simulink model "SLAMtester1"  (R2014a)
settings: Solver=FixedStepDiscrete  StartTime=0.0  StopTime=inf  FixedStep=.1  RelTol=1e-3
undefined symbols (not defined in the file): Com1, Com2, Com3, Com4, RGB24, standard
libraries: xpcseriallib x10, speedgoatlib_IO102 x6, slrtlib x4, xpcvideousblib x2, xpcvideoutillib x2, speedgoatlib x1
(part 1 of 2)
settings Model: BufferReuse=off  Creator=wildcat  LastModifiedBy=Villanova ASV
settings SolverCC: EnableConcurrentExecution=on
settings DataIOCC: SignalLoggingSaveFormat=ModelDataLogs
settings OptimizationCC: BlockReduction=off  OptimizeBlockIOStorage=off  BufferReuse=off  GlobalBufferReuse=off  ExpressionFolding=off  LocalBlockOutputs=off
settings DebuggingCC: UnderspecifiedInitializationDetection=Classic  StateNameClashWarn=warning
settings HardwareCC: ProdIntDivRoundTo=Zero  ProdEndianess=LittleEndian  ProdHWDeviceType=Generic->32-bit x86 compatible
settings RTWCC: SystemTargetFile=slrt.tlc  TemplateMakefile=slrt_default_tmf  Description=Simulink Real-Time  ProcessScript=slrt_make_rtw_hook  RTWCompilerOptimization=On
settings SimulinkRealTimeCC: GeneratePreprocessorConditionals=Disable all  EnableShiftOperators=on

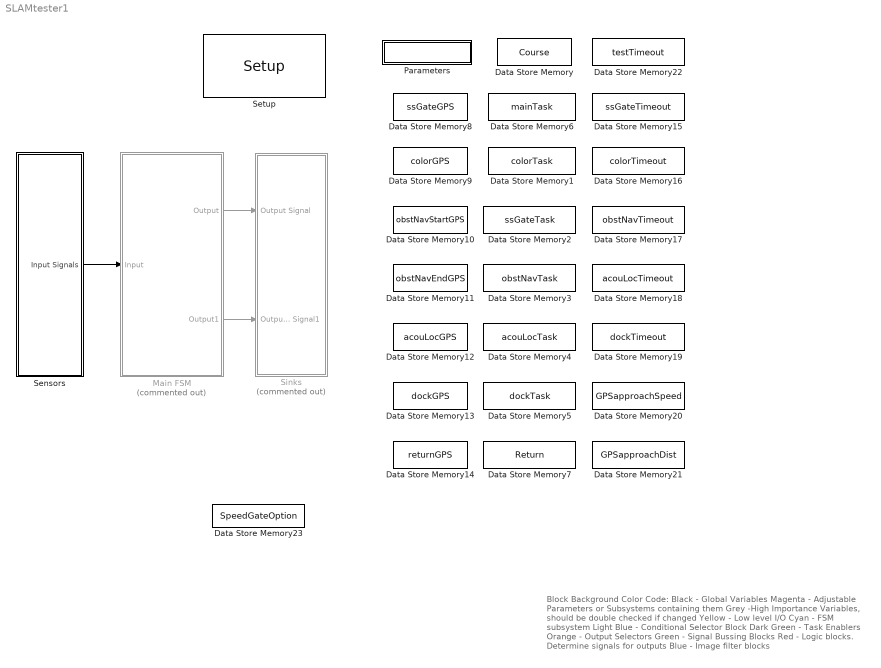
== system SLAMtester1 ==
  note: Block Background Color Code:
      | Black - Global Variables
      | Magenta - Adjustable Parameters or Subsystems containing them
      | Grey -High Importance Variables, should be double checked if changed
      | Yellow - Low level I/O
      | Cyan - FSM subsystem
      | Light Blue - Conditional Selector Block
      | Dark Green - Task Enablers
      | Orange - Output Selectors
      | Green - Signal Bussing Blocks
      | Red - Logic blocks. Determine signals for outputs
      | Blue - Image filter blocks
  Data Store Memory : DataStoreMemory  DataStoreName=Course  ReadBeforeWriteMsg=warning  WriteAfterWriteMsg=warning  WriteAfterReadMsg=warning
  Data Store Memory1 : DataStoreMemory  DataStoreName=colorTask  ReadBeforeWriteMsg=warning  WriteAfterWriteMsg=warning  WriteAfterReadMsg=warning  InitialValue=zeros(1,8)
  Data Store Memory10 : DataStoreMemory  DataStoreName=obstNavStartGPS  ReadBeforeWriteMsg=warning  WriteAfterWriteMsg=warning  WriteAfterReadMsg=warning  InitialValue=zeros(1,2)
  Data Store Memory11 : DataStoreMemory  DataStoreName=obstNavEndGPS  ReadBeforeWriteMsg=warning  WriteAfterWriteMsg=warning  WriteAfterReadMsg=warning  InitialValue=zeros(1,2)
  Data Store Memory12 : DataStoreMemory  DataStoreName=acouLocGPS  ReadBeforeWriteMsg=warning  WriteAfterWriteMsg=warning  WriteAfterReadMsg=warning  InitialValue=zeros(1,2)
  Data Store Memory13 : DataStoreMemory  DataStoreName=dockGPS  ReadBeforeWriteMsg=warning  WriteAfterWriteMsg=warning  WriteAfterReadMsg=warning  InitialValue=zeros(1,2)
  Data Store Memory14 : DataStoreMemory  DataStoreName=returnGPS  ReadBeforeWriteMsg=warning  WriteAfterWriteMsg=warning  WriteAfterReadMsg=warning  InitialValue=zeros(1,2)
  Data Store Memory15 : DataStoreMemory  DataStoreName=ssGateTimeout  ReadBeforeWriteMsg=warning  WriteAfterWriteMsg=warning  WriteAfterReadMsg=warning
  Data Store Memory16 : DataStoreMemory  DataStoreName=colorTimeout  ReadBeforeWriteMsg=warning  WriteAfterWriteMsg=warning  WriteAfterReadMsg=warning
  Data Store Memory17 : DataStoreMemory  DataStoreName=obstNavTimeout  ReadBeforeWriteMsg=warning  WriteAfterWriteMsg=warning  WriteAfterReadMsg=warning
  Data Store Memory18 : DataStoreMemory  DataStoreName=acouLocTimeout  ReadBeforeWriteMsg=warning  WriteAfterWriteMsg=warning  WriteAfterReadMsg=warning
  Data Store Memory19 : DataStoreMemory  DataStoreName=dockTimeout  ReadBeforeWriteMsg=warning  WriteAfterWriteMsg=warning  WriteAfterReadMsg=warning
  Data Store Memory2 : DataStoreMemory  DataStoreName=ssGateTask  ReadBeforeWriteMsg=warning  WriteAfterWriteMsg=warning  WriteAfterReadMsg=warning  InitialValue=zeros(1,8)
  Data Store Memory20 : DataStoreMemory  DataStoreName=GPSapproachSpeed  ReadBeforeWriteMsg=warning  WriteAfterWriteMsg=warning  WriteAfterReadMsg=warning
  Data Store Memory21 : DataStoreMemory  DataStoreName=GPSapproachDist  ReadBeforeWriteMsg=warning  WriteAfterWriteMsg=warning  WriteAfterReadMsg=warning
  Data Store Memory22 : DataStoreMemory  DataStoreName=testTimeout  ReadBeforeWriteMsg=warning  WriteAfterWriteMsg=warning  WriteAfterReadMsg=warning
  Data Store Memory23 : DataStoreMemory  DataStoreName=SpeedGateOption  ReadBeforeWriteMsg=warning  WriteAfterWriteMsg=warning  WriteAfterReadMsg=warning  InitialValue=zeros(1,8)
  Data Store Memory3 : DataStoreMemory  DataStoreName=obstNavTask  ReadBeforeWriteMsg=warning  WriteAfterWriteMsg=warning  WriteAfterReadMsg=warning  InitialValue=zeros(1,8)
  Data Store Memory4 : DataStoreMemory  DataStoreName=acouLocTask  ReadBeforeWriteMsg=warning  WriteAfterWriteMsg=warning  WriteAfterReadMsg=warning  InitialValue=zeros(1,8)
  Data Store Memory5 : DataStoreMemory  DataStoreName=dockTask  ReadBeforeWriteMsg=warning  WriteAfterWriteMsg=warning  WriteAfterReadMsg=warning  InitialValue=zeros(1,8)
  Data Store Memory6 : DataStoreMemory  DataStoreName=mainTask  ReadBeforeWriteMsg=warning  WriteAfterWriteMsg=warning  WriteAfterReadMsg=warning  InitialValue=zeros(1,8)
  Data Store Memory7 : DataStoreMemory  DataStoreName=Return  ReadBeforeWriteMsg=warning  WriteAfterWriteMsg=warning  WriteAfterReadMsg=warning  InitialValue=zeros(1,8)
  Data Store Memory8 : DataStoreMemory  DataStoreName=ssGateGPS  ReadBeforeWriteMsg=warning  WriteAfterWriteMsg=warning  WriteAfterReadMsg=warning  InitialValue=zeros(1,2)
  Data Store Memory9 : DataStoreMemory  DataStoreName=colorGPS  ReadBeforeWriteMsg=warning  WriteAfterWriteMsg=warning  WriteAfterReadMsg=warning  InitialValue=zeros(1,2)
  Main FSM : Subsystem  Commented=on
  Parameters : Subsystem
  Sensors : Subsystem
  Setup : speedgoatlib_IO102/Setup  group=Analog input setup  id=1  range=+-5V  cal=off  pciSlot=-1  adChannelMode=Multiple-channel (enter number of channels below)  adChannel=16  adCoupling=Differential  daChannel=[1,2,3,4]  daReset=[1]  daInitValue=[0]  diChannel=[1,2,3,4,5,6,7,8]  doChannel=[1,2,3,4,5,6,7,8]  doReset=[1]  doInitValue=[0]
  Sinks : Subsystem  Commented=on
  wires:
  Main FSM/1(Output) -> Sinks/1(Output Signal)
  Sensors/1(Input Signals) -> Main FSM/1(Input)
  Main FSM/2(Output1) -> Sinks/2(Output Signal1)

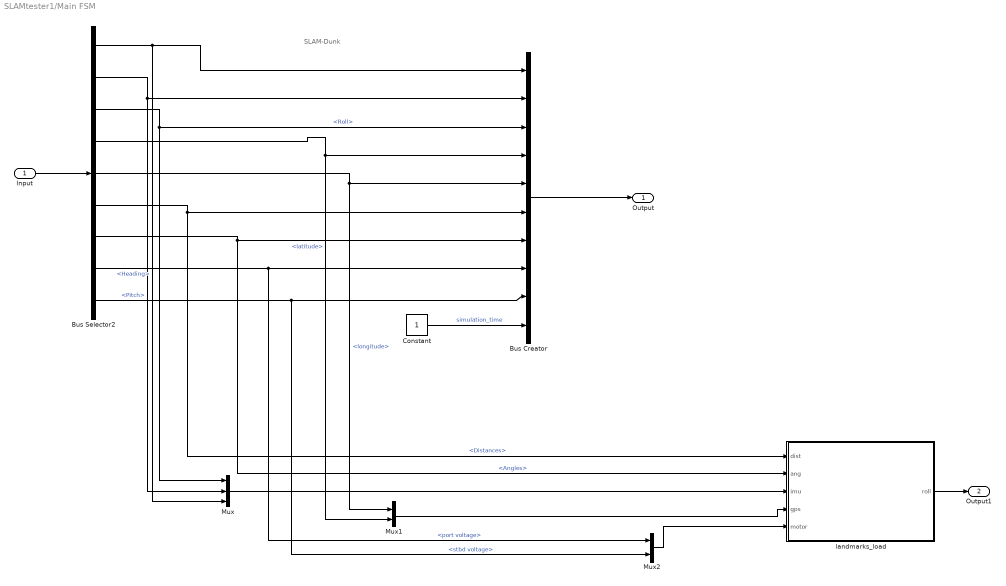
== system SLAMtester1/Main FSM ==
  note: SLAM-Dunk
  Input : Inport
  Bus Creator : BusCreator  Inputs=10
  Bus Selector2 : BusSelector  OutputSignals=Sensors.Serial In.Compass.Heading,Sensors.Serial In.Compass.Pitch,Sensors.Serial In.Compass.Roll,Sensors.Serial In.GPS.latitude,Sensors.Serial In.GPS.longitude,Sensors.Serial In.Landmarks.Distances,Sensors.Serial In.Landmarks.Angles,Sensors.thrusters.port voltage,Sensors.thrusters.stbd voltage
  Constant : Constant
  Mux : Mux  Inputs=3
  Mux1 : Mux  Inputs=2
  Mux2 : Mux  Inputs=2
  landmarks_load : MATLAB Function  TreatAsAtomicUnit=on
  Output : Outport
  Output1 : Outport  Port=2
  wires:
  Input/1 -> Bus Selector2/1
  Bus Selector2/1 -> Mux/3, Bus Creator/1  "<Heading>"
  Bus Selector2/2 -> Mux/2, Bus Creator/2  "<Pitch>"
  Bus Selector2/3 -> Mux/1, Bus Creator/3  "<Roll>"
  Bus Selector2/4 -> Mux1/2, Bus Creator/4  "<latitude>"
  Bus Selector2/5 -> Mux1/1, Bus Creator/5  "<longitude>"
  Bus Selector2/6 -> landmarks_load/1(dist), Bus Creator/6  "<Distances>"
  Bus Selector2/7 -> landmarks_load/2(ang), Bus Creator/7  "<Angles>"
  Bus Selector2/8 -> Mux2/1, Bus Creator/8  "<port voltage>"
  Bus Selector2/9 -> Mux2/2, Bus Creator/9  "<stbd voltage>"
  Bus Creator/1 -> Output/1
  Constant/1 -> Bus Creator/10  "simulation_time"
  Mux/1 -> landmarks_load/3(imu)
  Mux1/1 -> landmarks_load/4(gps)
  landmarks_load/1(roll) -> Output1/1
  Mux2/1 -> landmarks_load/5(motor)

== system SLAMtester1/Parameters ==
  note: Course options are:
      | A, B and
      | otherwise (for testing,
      |  must be one character)
  CourseName : Constant  Value=uint8('T')  VectorParams1D=off
  GPS Points : Subsystem
  Task Options : Subsystem
  Task Selector : Subsystem
  Timeouts and Constants : Subsystem
  Write : DataStoreWrite  DataStoreName=Course
  wires:
  CourseName/1 -> Write/1

== system SLAMtester1/Sensors ==
  Analog In : Subsystem  Commented=on
  Bus Creator : BusCreator  Inputs=3
  Bus Creator1 : BusCreator  Inputs=2
  Digital In : Subsystem
  Serial In : Subsystem
  Video In : Subsystem
  Input Signals : Outport
  wires:
  Serial In/1(Serial In) -> Bus Creator/1
  Digital In/1(Digital In) -> Bus Creator/3
  Video In/1(RGB image) -> Bus Creator1/2
  Bus Creator/1 -> Bus Creator1/1  "Sensors"
  Bus Creator1/1 -> Input Signals/1
  Analog In/1(analog in) -> Bus Creator/2

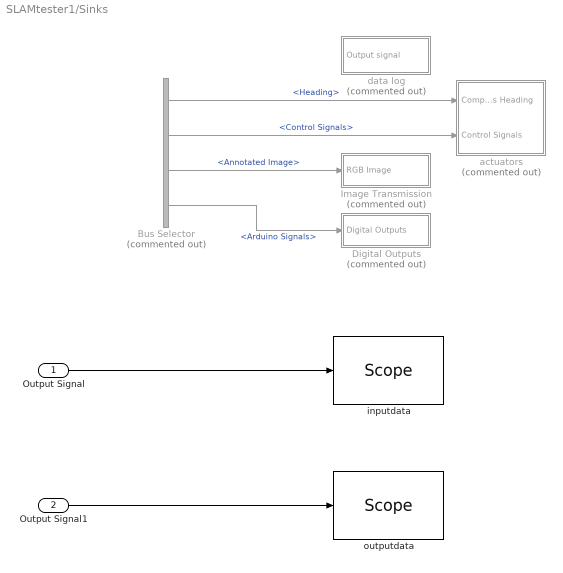
== system SLAMtester1/Sinks ==
  Output Signal : Inport
  Output Signal1 : Inport  Port=2
  Bus Selector : BusSelector  Commented=on  OutputSignals=Sensors.Serial In.Compass.Heading,Outputs.Control Signals,Outputs.Annotated Image,Outputs.Control Signals.Arduino Signals
  Digital Outputs : Subsystem  Commented=on
  Image Transmission : Subsystem  Commented=on
  actuators : Subsystem  Commented=on
  data log : Subsystem  Commented=on
  inputdata : slrtlib/Displays and Logging/Scope   scopeno=2  scopetype=File  autostart=on  viewmode=Graphical redraw  formatstr='%15.6f'  grid=on  ylimits=[0,0]  nosamples=10*5*600  noprepostsamples=0  interleave=1  triggermode=FreeRun  triggersignal=1  trigsignalfromport=off  triggerlevel=0.0  triggerslope=Either  triggerscope=1  triggersample=0  filename=landmark.dat  mode=Lazy  writesize=512  autorestart=off  dynamicfilemode=off  maxwritefilesize=512*1024^2
  outputdata : slrtlib/Displays and Logging/Scope   scopeno=3  scopetype=File  autostart=on  viewmode=Graphical redraw  formatstr='%15.6f'  grid=on  ylimits=[0,0]  nosamples=10*5*600  noprepostsamples=0  interleave=1  triggermode=FreeRun  triggersignal=1  trigsignalfromport=off  triggerlevel=0.0  triggerslope=Either  triggerscope=1  triggersample=0  filename=particle.dat  mode=Lazy  writesize=512  autorestart=off  dynamicfilemode=off  maxwritefilesize=512*1024^2
  wires:
  Bus Selector/2 -> actuators/2(Control Signals)  "<Control Signals>"
  Bus Selector/3 -> Image Transmission/1(RGB Image)  "<Annotated Image>"
  Bus Selector/1 -> actuators/1(Compass Heading)  "<Heading>"
  Output Signal/1 -> inputdata/1
  Bus Selector/4 -> Digital Outputs/1(Digital Outputs)  "<Arduino Signals>"
  Output Signal1/1 -> outputdata/1

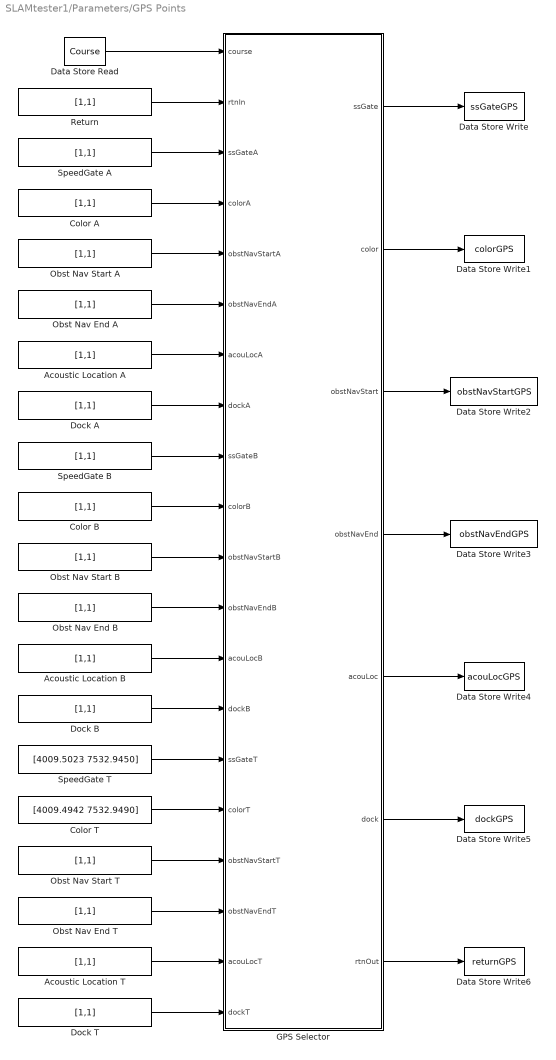
== system SLAMtester1/Parameters/GPS Points ==
  Acoustic Location A : Constant  Value=[1,1]  SampleTime=0.1
  Acoustic Location B : Constant  Value=[1,1]  SampleTime=0.1
  Acoustic Location T : Constant  Value=[1,1]  SampleTime=0.1
  Color A : Constant  Value=[1,1]  SampleTime=0.1
  Color B : Constant  Value=[1,1]  SampleTime=0.1
  Color T : Constant  Value=[4009.4942 7532.9490]  SampleTime=0.1
  Data Store Read : DataStoreRead  DialogController=Simulink.DDGSource  DataStoreName=Course  SampleTime=0.1
  Data Store Write : DataStoreWrite  DialogController=Simulink.DDGSource  DataStoreName=ssGateGPS
  Data Store Write1 : DataStoreWrite  DataStoreName=colorGPS
  Data Store Write2 : DataStoreWrite  DataStoreName=obstNavStartGPS
  Data Store Write3 : DataStoreWrite  DataStoreName=obstNavEndGPS
  Data Store Write4 : DataStoreWrite  DataStoreName=acouLocGPS
  Data Store Write5 : DataStoreWrite  DataStoreName=dockGPS
  Data Store Write6 : DataStoreWrite  DataStoreName=returnGPS
  Dock A : Constant  Value=[1,1]  SampleTime=0.1
  Dock B : Constant  Value=[1,1]  SampleTime=0.1
  Dock T : Constant  Value=[1,1]  SampleTime=0.1
  GPS Selector : MATLAB Function  TreatAsAtomicUnit=on
  Obst Nav End A : Constant  Value=[1,1]  SampleTime=0.1
  Obst Nav End B : Constant  Value=[1,1]  SampleTime=0.1
  Obst Nav End T : Constant  Value=[1,1]  SampleTime=0.1
  Obst Nav Start A : Constant  Value=[1,1]  SampleTime=0.1
  Obst Nav Start B : Constant  Value=[1,1]  SampleTime=0.1
  Obst Nav Start T : Constant  Value=[1,1]  SampleTime=0.1
  Return : Constant  Value=[1,1]  SampleTime=0.1
  SpeedGate A : Constant  Value=[1,1]  SampleTime=0.1
  SpeedGate B : Constant  Value=[1,1]  SampleTime=0.1
  SpeedGate T : Constant  Value=[4009.5023 7532.9450]  SampleTime=0.1
  wires:
  Data Store Read/1 -> GPS Selector/1(course)
  Return/1 -> GPS Selector/2(rtnIn)
  SpeedGate A/1 -> GPS Selector/3(ssGateA)
  Color A/1 -> GPS Selector/4(colorA)
  Obst Nav Start A/1 -> GPS Selector/5(obstNavStartA)
  Obst Nav End A/1 -> GPS Selector/6(obstNavEndA)
  SpeedGate T/1 -> GPS Selector/15(ssGateT)
  Acoustic Location T/1 -> GPS Selector/19(acouLocT)
  Color T/1 -> GPS Selector/16(colorT)
  Dock A/1 -> GPS Selector/8(dockA)
  Dock T/1 -> GPS Selector/20(dockT)
  Obst Nav End T/1 -> GPS Selector/18(obstNavEndT)
  Obst Nav Start T/1 -> GPS Selector/17(obstNavStartT)
  Obst Nav Start B/1 -> GPS Selector/11(obstNavStartB)
  Obst Nav End B/1 -> GPS Selector/12(obstNavEndB)
  Acoustic Location A/1 -> GPS Selector/7(acouLocA)
  Acoustic Location B/1 -> GPS Selector/13(acouLocB)
  Dock B/1 -> GPS Selector/14(dockB)
  SpeedGate B/1 -> GPS Selector/9(ssGateB)
  Color B/1 -> GPS Selector/10(colorB)
  GPS Selector/1(ssGate) -> Data Store Write/1
  GPS Selector/2(color) -> Data Store Write1/1
  GPS Selector/3(obstNavStart) -> Data Store Write2/1
  GPS Selector/4(obstNavEnd) -> Data Store Write3/1
  GPS Selector/5(acouLoc) -> Data Store Write4/1
  GPS Selector/6(dock) -> Data Store Write5/1
  GPS Selector/7(rtnOut) -> Data Store Write6/1

== system SLAMtester1/Parameters/Task Options ==
  note: otherwise skips and treats as buoys
  note: Options:
      | Shotgun
      | GPS
  note: *note*
      | left course generally has issues
      | treating the gates as buoys.
      | tends to find right course gates
      | and head towards them
  Fix length : MATLAB Function  TreatAsAtomicUnit=on
  Speed Gate Option : Constant  Value=uint8('Shotgun')
  Write : DataStoreWrite  DataStoreName=SpeedGateOption
  wires:
  Speed Gate Option/1 -> Fix length/1(selection)
  Fix length/1(adjusted) -> Write/1

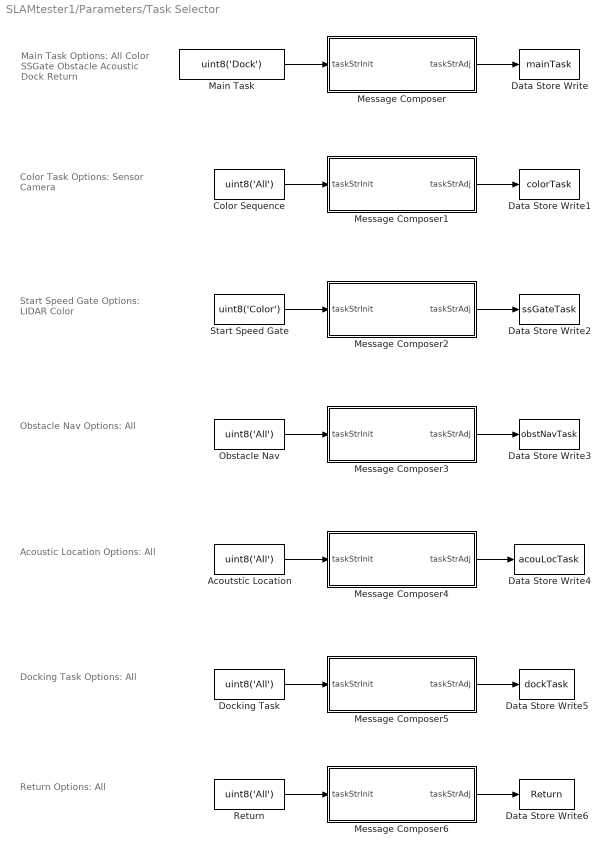
== system SLAMtester1/Parameters/Task Selector ==
  note: Docking Task Options:
      | All
  note: Acoustic Location Options:
      | All
  note: Obstacle Nav Options:
      | All
  note: Start Speed Gate Options:
      | LIDAR
      | Color
  note: Color Task Options:
      | Sensor
      | Camera
  note: Main Task Options:
      | All
      | Color
      | SSGate
      | Obstacle
      | Acoustic
      | Dock
      | Return
  note: Return Options:
      | All
  Acoutstic Location : Constant  Value=uint8('All')  SampleTime=0.1
  Color Sequence : Constant  Value=uint8('All')  SampleTime=0.1
  Data Store Write : DataStoreWrite  DataStoreName=mainTask
  Data Store Write1 : DataStoreWrite  DialogController=Simulink.DDGSource  DataStoreName=colorTask
  Data Store Write2 : DataStoreWrite  DataStoreName=ssGateTask
  Data Store Write3 : DataStoreWrite  DataStoreName=obstNavTask
  Data Store Write4 : DataStoreWrite  DataStoreName=acouLocTask
  Data Store Write5 : DataStoreWrite  DataStoreName=dockTask
  Data Store Write6 : DataStoreWrite  DataStoreName=Return
  Docking Task : Constant  Value=uint8('All')  SampleTime=0.1
  Main Task : Constant  Value=uint8('Dock')  SampleTime=0.1
  Message Composer : MATLAB Function  TreatAsAtomicUnit=on
  Message Composer1 : MATLAB Function  TreatAsAtomicUnit=on
  Message Composer2 : MATLAB Function  TreatAsAtomicUnit=on
  Message Composer3 : MATLAB Function  TreatAsAtomicUnit=on
  Message Composer4 : MATLAB Function  TreatAsAtomicUnit=on
  Message Composer5 : MATLAB Function  TreatAsAtomicUnit=on
  Message Composer6 : MATLAB Function  TreatAsAtomicUnit=on
  Obstacle Nav : Constant  Value=uint8('All')  SampleTime=0.1
  Return : Constant  Value=uint8('All')  SampleTime=0.1
  Start Speed Gate : Constant  Value=uint8('Color')  SampleTime=0.1
  wires:
  Main Task/1 -> Message Composer/1(taskStrInit)
  Message Composer/1(taskStrAdj) -> Data Store Write/1
  Color Sequence/1 -> Message Composer1/1(taskStrInit)
  Message Composer1/1(taskStrAdj) -> Data Store Write1/1
  Start Speed Gate/1 -> Message Composer2/1(taskStrInit)
  Message Composer2/1(taskStrAdj) -> Data Store Write2/1
  Obstacle Nav/1 -> Message Composer3/1(taskStrInit)
  Message Composer3/1(taskStrAdj) -> Data Store Write3/1
  Acoutstic Location/1 -> Message Composer4/1(taskStrInit)
  Message Composer4/1(taskStrAdj) -> Data Store Write4/1
  Docking Task/1 -> Message Composer5/1(taskStrInit)
  Message Composer5/1(taskStrAdj) -> Data Store Write5/1
  Return/1 -> Message Composer6/1(taskStrInit)
  Message Composer6/1(taskStrAdj) -> Data Store Write6/1

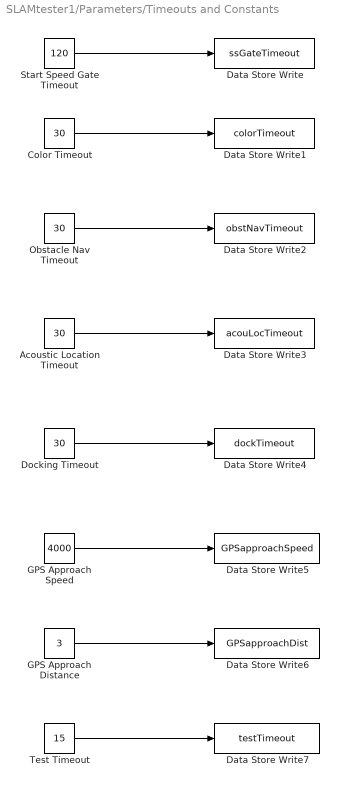
== system SLAMtester1/Parameters/Timeouts and Constants ==
  Acoustic Location Timeout : Constant  Value=30  SampleTime=0.1
  Color Timeout : Constant  Value=30  SampleTime=0.1
  Data Store Write : DataStoreWrite  DataStoreName=ssGateTimeout
  Data Store Write1 : DataStoreWrite  DataStoreName=colorTimeout
  Data Store Write2 : DataStoreWrite  DataStoreName=obstNavTimeout
  Data Store Write3 : DataStoreWrite  DataStoreName=acouLocTimeout
  Data Store Write4 : DataStoreWrite  DataStoreName=dockTimeout
  Data Store Write5 : DataStoreWrite  DataStoreName=GPSapproachSpeed
  Data Store Write6 : DataStoreWrite  DataStoreName=GPSapproachDist
  Data Store Write7 : DataStoreWrite  DataStoreName=testTimeout
  Docking Timeout : Constant  Value=30  SampleTime=0.1
  GPS Approach Distance : Constant  Value=3  SampleTime=0.1
  GPS Approach Speed : Constant  Value=4000  SampleTime=0.1
  Obstacle Nav Timeout : Constant  Value=30  SampleTime=0.1
  Start Speed Gate Timeout : Constant  Value=120  SampleTime=0.1
  Test Timeout : Constant  Value=15  SampleTime=0.1
  wires:
  Start Speed Gate Timeout/1 -> Data Store Write/1
  Color Timeout/1 -> Data Store Write1/1
  Acoustic Location Timeout/1 -> Data Store Write3/1
  Docking Timeout/1 -> Data Store Write4/1
  GPS Approach Speed/1 -> Data Store Write5/1
  GPS Approach Distance/1 -> Data Store Write6/1
  Obstacle Nav Timeout/1 -> Data Store Write2/1
  Test Timeout/1 -> Data Store Write7/1

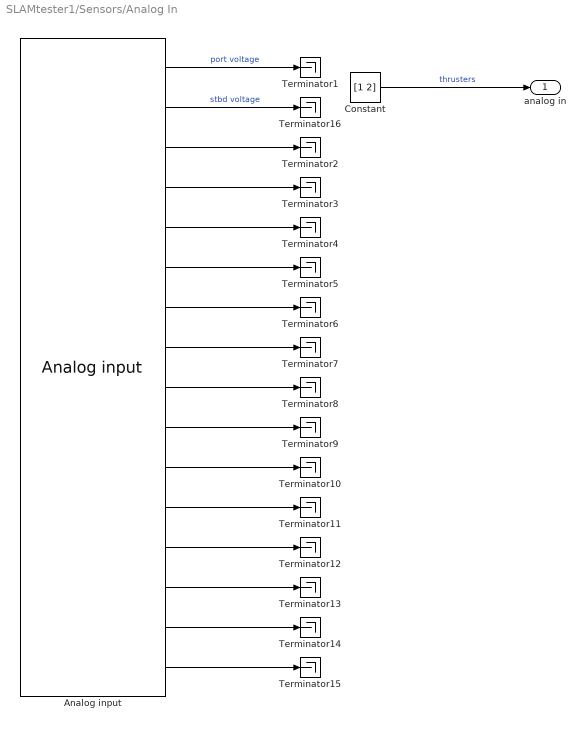
== system SLAMtester1/Sensors/Analog In ==
  Analog input : speedgoatlib_IO102/Analog input  id=1  channels=[1,2,3,4,5,6,7,8,9,10,11,12,13,14,15,16]  range=2  high_voltage=off  adCoupling=1  ts=-1  pciSlot=-1
  Constant : Constant  Value=[1 2]
  Terminator{1..16} (16 alike) : Terminator
  analog in : Outport
  wires:
  Analog input/1 -> Terminator1/1  "port voltage"
  Analog input/2 -> Terminator16/1  "stbd voltage"
  Analog input/3 -> Terminator2/1
  Analog input/4 -> Terminator3/1
  Analog input/5 -> Terminator4/1
  Analog input/6 -> Terminator5/1
  Analog input/7 -> Terminator6/1
  Analog input/8 -> Terminator7/1
  Analog input/9 -> Terminator8/1
  Analog input/10 -> Terminator9/1
  Analog input/11 -> Terminator10/1
  Analog input/12 -> Terminator11/1
  Analog input/13 -> Terminator12/1
  Analog input/14 -> Terminator13/1
  Analog input/15 -> Terminator14/1
  Analog input/16 -> Terminator15/1
  Constant/1 -> analog in/1  "thrusters"

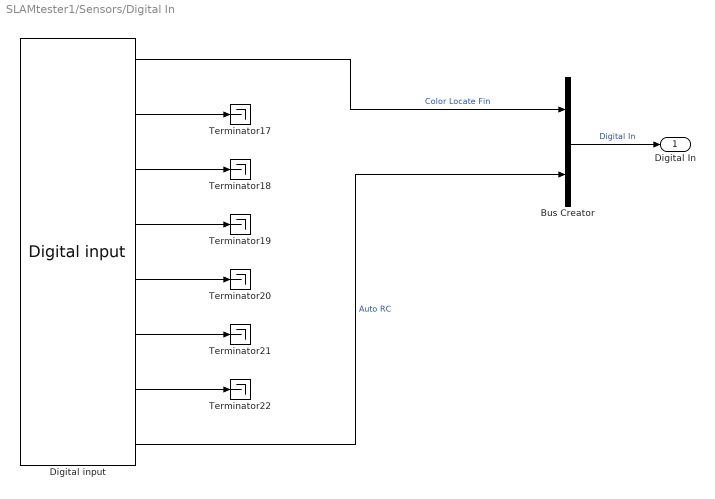
== system SLAMtester1/Sensors/Digital In ==
  Bus Creator : BusCreator  Inputs=2
  Digital input : speedgoatlib_IO102/Digital input  id=1  channels=[1,2,3,4,5,6,7,8]  ts=0.1  pciSlot=-1
  Terminator{17..22} (6 alike) : Terminator
  Digital In : Outport
  wires:
  Bus Creator/1 -> Digital In/1  "Digital In"
  Digital input/8 -> Bus Creator/2  "Auto RC"
  Digital input/2 -> Terminator17/1
  Digital input/3 -> Terminator18/1
  Digital input/4 -> Terminator19/1
  Digital input/5 -> Terminator20/1
  Digital input/6 -> Terminator21/1
  Digital input/7 -> Terminator22/1
  Digital input/1 -> Bus Creator/1  "Color Locate Fin"

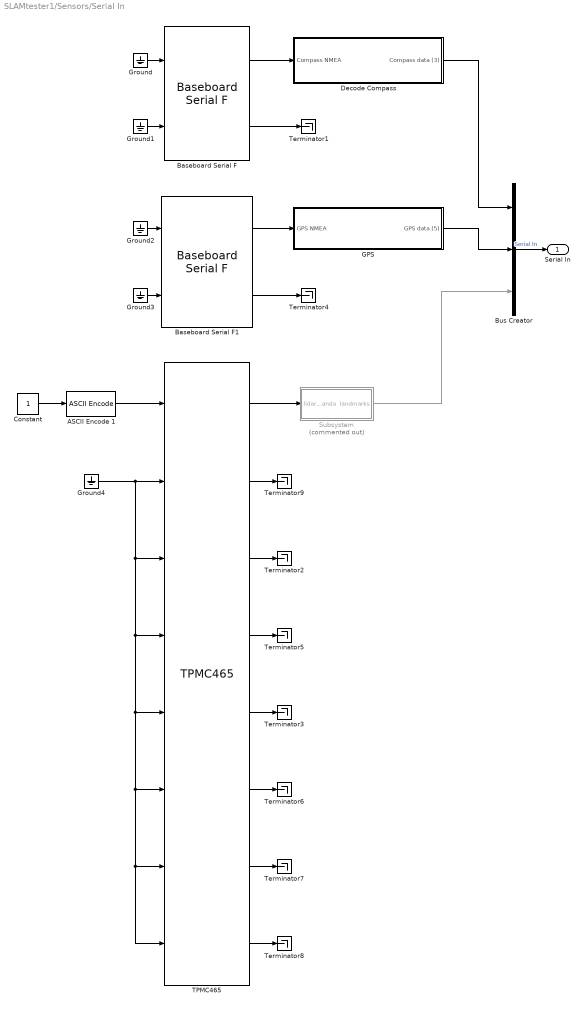
== system SLAMtester1/Sensors/Serial In ==
  " GPS" : Subsystem
  ASCII Encode 1 : xpcseriallib/ASCII Encode   format=SGTask:%d\r\n  nvars=1  maxlength=128  vartypes={ 'double' }
  Baseboard Serial F : xpcseriallib/Mainboard/Baseboard Serial F  group=Basic Setup  port=2  irqnum=4  saddr1=0x3f8  saddr2=0x3e8  config=Com1/Com3  baud1=19200  parity1=None  ndata1=8  nstop1=1  fifomode1=64 deep  rlevel1=half full  automode1=on  xmtfifosize1=1024  xmtdatatype1=8 bit uint null terminated  rcvfifosize1=1024  baud2=115200  parity2=None  ndata2=8  nstop2=1  fifomode2=64 deep  rlevel2=half full  automode2=on  xmtfifosize2=1024  xmtdatatype2=8 bit uint null terminated  rcvfifosize2=1024
  Baseboard Serial F1 : xpcseriallib/Mainboard/Baseboard Serial F  group=Basic Setup  port=2  irqnum=4  saddr1=0x3f8  saddr2=0x3e8  config=Com2/Com4  baud1=19200  parity1=None  ndata1=8  nstop1=1  fifomode1=64 deep  rlevel1=half full  automode1=on  xmtfifosize1=1024  xmtdatatype1=8 bit uint null terminated  rcvfifosize1=1024  baud2=115200  parity2=None  ndata2=8  nstop2=1  fifomode2=64 deep  rlevel2=half full  automode2=on  xmtfifosize2=1024  xmtdatatype2=8 bit uint null terminated  rcvfifosize2=1024
  Bus Creator : BusCreator  Inputs=3
  Constant : Constant  SampleTime=0.1
  Decode Compass : Subsystem
  Ground{,1..4} (5 alike) : Ground
  Subsystem : Subsystem  Commented=on
  TPMC465 : speedgoatlib/IO504/TPMC465  group=Basic Setup  port=1  irqnum=9  slot=-1  transceiver1=RS232 (max 921.6kb/s)  standard1=on  baud1=115200  bauddivisor1=1  sampling1=16x (standard)  prescale1=off  parity1=Even  ndata1=7  nstop1=1  rlevel1=quarter full (16)  hwmode1=none  swmode1=none  xonchar1=17  xoffchar1=19  rs485auto1=off  rs485delay1=0  xmtfifosize1=1024  xmtdatatype1=8 bit uint null terminated  rcvfifosize1=1024  transceiver2=RS232 (max 921.6kb/s)  standard2=on  baud2=115200  bauddivisor2=1  sampling2=16x (standard)  prescale2=off  parity2=None  ndata2=8  nstop2=1  rlevel2=half full (32)  hwmode2=none  swmode2=none  xonchar2=17  xoffchar2=19  rs485auto2=off  rs485delay2=0  xmtfifosize2=1024  xmtdatatype2=8 bit uint null terminated  rcvfifosize2=1024  transceiver3=RS232 (max 921.6kb/s)  standard3=on  baud3=115200  bauddivisor3=1  sampling3=16x (standard)  prescale3=off  parity3=None  ndata3=8  nstop3=1  rlevel3=half full (32)  hwmode3=none  swmode3=none  xonchar3=17  xoffchar3=19  rs485auto3=off  rs485delay3=0  xmtfifosize3=1024  xmtdatatype3=8 bit uint null terminated  rcvfifosize3=1024  transceiver4=RS232 (max 921.6kb/s)  standard4=on  baud4=115200  bauddivisor4=1  sampling4=16x (standard)  prescale4=off  parity4=None  ndata4=8  nstop4=1  rlevel4=half full (32)  hwmode4=none  swmode4=none  xonchar4=17  xoffchar4=19  rs485auto4=off  rs485delay4=0  xmtfifosize4=1024  xmtdatatype4=8 bit uint null terminated  rcvfifosize4=1024  transceiver5=RS232 (max 921.6kb/s)  standard5=on  baud5=115200  bauddivisor5=1  sampling5=16x (standard)  prescale5=off  parity5=None  ndata5=8  nstop5=1  rlevel5=1  hwmode5=none  swmode5=none  xonchar5=17  xoffchar5=19  rs485auto5=off  rs485delay5=0  xmtfifosize5=1024  xmtdatatype5=8 bit uint null terminated  rcvfifosize5=1024  transceiver6=RS232 (max 921.6kb/s)  standard6=on  baud6=115200  bauddivisor6=1  sampling6=16x (standard)  prescale6=off  parity6=None  ndata6=8  nstop6=1  rlevel6=1  hwmode6=none  swmode6=none  xonchar6=17  xoffchar6=19  rs485auto6=off  rs485delay6=0  xmtfifosize6=1024  xmtdatatype6=8 bit uint null terminated  rcvfifosize6=1024  transceiver7=RS232 (max 921.6kb/s)  standard7=on  baud7=115200  bauddivisor7=1  sampling7=16x (standard)  prescale7=off  parity7=None  ndata7=8  nstop7=1  rlevel7=1  hwmode7=none  swmode7=none  xonchar7=17  xoffchar7=19  rs485auto7=off  rs485delay7=0  xmtfifosize7=1024  xmtdatatype7=8 bit uint null terminated  rcvfifosize7=1024  transceiver8=RS232 (max 921.6kb/s)  standard8=on  baud8=115200  bauddivisor8=1  sampling8=16x (standard)  prescale8=off  parity8=None  ndata8=8  nstop8=1  rlevel8=1  hwmode8=none  swmode8=none  xonchar8=17  xoffchar8=19  rs485auto8=off  rs485delay8=0  xmtfifosize8=1024  xmtdatatype8=8 bit uint null terminated  rcvfifosize8=1024
  Terminator{1..9} (9 alike) : Terminator
  Serial In : Outport
  wires:
  Decode Compass/1(Compass data (3)) -> Bus Creator/1
  " GPS"/1(GPS data (5)) -> Bus Creator/2
  Bus Creator/1 -> Serial In/1  "Serial In"
  Ground4/1 -> TPMC465/3, TPMC465/6, TPMC465/8, TPMC465/7, TPMC465/5, TPMC465/4, TPMC465/2
  TPMC465/6 -> Terminator6/1
  TPMC465/7 -> Terminator7/1
  TPMC465/8 -> Terminator8/1
  TPMC465/5 -> Terminator3/1
  Ground/1 -> Baseboard Serial F/1
  Ground1/1 -> Baseboard Serial F/2
  Baseboard Serial F/1 -> Decode Compass/1(Compass NMEA)
  Ground3/1 -> Baseboard Serial F1/2
  Ground2/1 -> Baseboard Serial F1/1
  Baseboard Serial F1/1 -> " GPS"/1(GPS NMEA)
  Baseboard Serial F/2 -> Terminator1/1
  Baseboard Serial F1/2 -> Terminator4/1
  TPMC465/4 -> Terminator5/1
  TPMC465/3 -> Terminator2/1
  ASCII Encode 1/1 -> TPMC465/1
  TPMC465/1 -> Subsystem/1(lidarPanda)
  Constant/1 -> ASCII Encode 1/1
  TPMC465/2 -> Terminator9/1
  Subsystem/1(landmarks) -> Bus Creator/3

== system SLAMtester1/Sensors/Video In ==
  Constant : Constant  Commented=on  Value=uint8(255*ones(480,640,3))
  From USB Video Device : xpcvideousblib/From USB Video Device  sconf=<Select a configuration>  paddr=-1  iwidth=640  iheight=480  fint=1/10  ffmt=Uncompressed  cfmt=RGB24 (8:8:8)  isig=One multidimensional signal  trigger=off  status=off  updateBlock=1
  USB Video Device List : xpcvideousblib/USB Video Device List  usb_search=on  ShowInLibBrowser=0
  RGB image : Outport
  wires:
  From USB Video Device/1 -> RGB image/1  "RGB Image"

== system SLAMtester1/Sinks/Digital Outputs ==
  Digital Outputs : Inport
  Bus Selector : BusSelector  OutputSignals=Ready to Read,Due Sample Start
  Digital output : speedgoatlib_IO102/Digital output  id=1  channels=[1,2,3,4,5,6,7,8]  ts=0.1  pciSlot=-1
  Ground : Ground
  wires:
  Digital Outputs/1 -> Bus Selector/1
  Bus Selector/1 -> Digital output/1  "<Ready to Read>"
  Bus Selector/2 -> Digital output/2  "<Due Sample Start>"
  Ground/1 -> Digital output/4, Digital output/8, Digital output/7, Digital output/6, Digital output/5, Digital output/3

== system SLAMtester1/Sinks/Image Transmission ==
  note: Image Transmission
  RGB Image : Inport
  Image Transmit : xpcvideoutillib/Image Transmit  ipAddress=255.255.255.255  ipPort=25000  localPort=-1  vblLen=on  maxpacket=40*1024  sampletime=-1
  Jpeg Compression1 : xpcvideoutillib/Jpeg Compression  quality=20  cspace=RGB  isig=One multidimensional signal  maxsize=640*480  length=on
  Rate Transition : RateTransition  OutPortSampleTime=1
  wires:
  Jpeg Compression1/1 -> Image Transmit/1
  Jpeg Compression1/2 -> Image Transmit/2
  Rate Transition/1 -> Jpeg Compression1/1
  RGB Image/1 -> Rate Transition/1

== system SLAMtester1/Sinks/actuators ==
  Compass Heading : Inport
  Control Signals : Inport  Port=2
  analog output : Subsystem
  digital output : Subsystem
  wires:
  Control Signals/1 -> digital output/1(Digital Out), analog output/2(Control Signals)
  Compass Heading/1 -> analog output/1(Compass Heading)

== system SLAMtester1/Sinks/data log ==
  note: need to play with the boat to figure out how this works properly
  Output signal : Inport
  "Scope " : slrtlib/Displays and Logging/Scope   scopeno=1  scopetype=File  autostart=on  viewmode=Graphical redraw  formatstr='%15.6f'  grid=on  ylimits=[0,0]  nosamples=250  noprepostsamples=0  interleave=1  triggermode=Signal triggering  triggersignal=1  trigsignalfromport=on  triggerlevel=1  triggerslope=Rising  triggerscope=1  triggersample=0  filename=data.dat  mode=Lazy  writesize=512  autorestart=off  dynamicfilemode=off  maxwritefilesize=512*1024^2
  wires:
  Output signal/1 -> ?

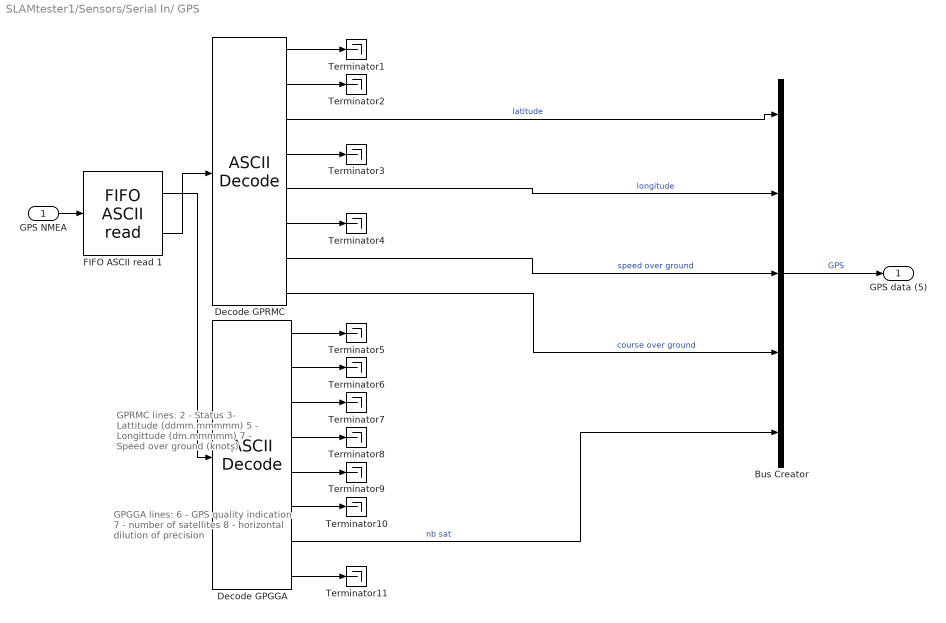
== system SLAMtester1/Sensors/Serial In/ GPS ==
  note: GPGGA lines:
      | 6 - GPS quality indication
      | 7 - number of satellites
      | 8 - horizontal dilution of precision
  note: GPRMC lines:
      | 2 - Status
      | 3- Lattitude (ddmm.mmmmm)
      | 5 - Longittude (dm.mmmmm)
      | 7 - Speed over ground (knots)
  GPS NMEA : Inport
  Bus Creator : BusCreator  Inputs=5
  Decode GPGGA : xpcseriallib/ASCII Decode   format=$GPGGA,%d,%f,%c%f,%c%f,%f,%f  nvars=8  vartypes={ }
  Decode GPRMC : xpcseriallib/ASCII Decode   format=$GPRMC,%f,%c%f,%c%f,%c%f,%f  nvars=8  vartypes={ }
  FIFO ASCII read 1 : xpcseriallib/FIFO ASCII read   header={'$GPGGA','$GPRMC'}  term=[13 10]  hold=Zero output if no new data  enable=off  maxsize=1024  outputtype=8 bit uint null terminated  sampletime=-1
  Terminator{1..11} (11 alike) : Terminator
  GPS data (5) : Outport
  wires:
  Decode GPRMC/1 -> Terminator1/1
  Decode GPRMC/7 -> Bus Creator/3  "speed over ground"
  Decode GPRMC/5 -> Bus Creator/2  "longitude"
  Decode GPRMC/3 -> Bus Creator/1  "latitude"
  GPS NMEA/1 -> FIFO ASCII read 1/1
  FIFO ASCII read 1/1 -> Decode GPGGA/1
  FIFO ASCII read 1/2 -> Decode GPRMC/1
  Decode GPRMC/8 -> Bus Creator/4  "course over ground"
  Decode GPGGA/7 -> Bus Creator/5  "nb sat"
  Decode GPRMC/2 -> Terminator2/1
  Decode GPRMC/4 -> Terminator3/1
  Decode GPRMC/6 -> Terminator4/1
  Decode GPGGA/1 -> Terminator5/1
  Decode GPGGA/2 -> Terminator6/1
  Decode GPGGA/3 -> Terminator7/1
  Decode GPGGA/4 -> Terminator8/1
  Decode GPGGA/5 -> Terminator9/1
  Decode GPGGA/6 -> Terminator10/1
  Decode GPGGA/8 -> Terminator11/1
  Bus Creator/1 -> GPS data (5)/1  "GPS"

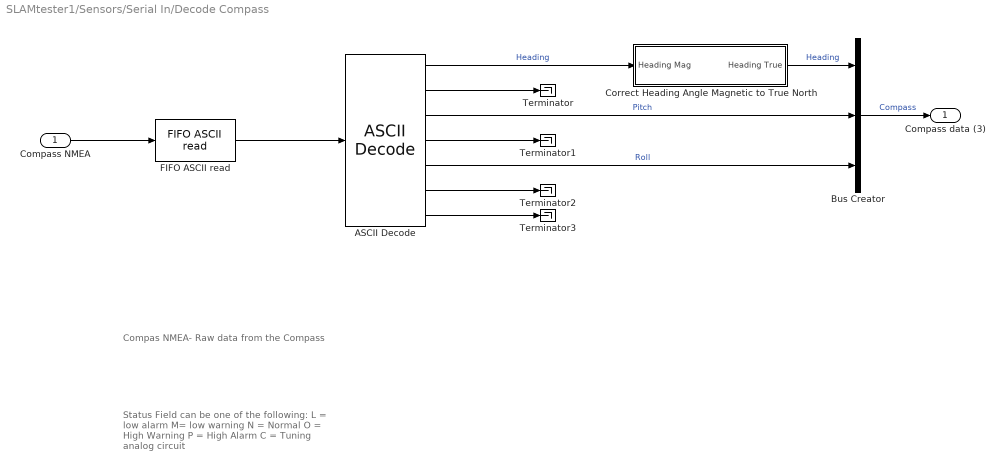
== system SLAMtester1/Sensors/Serial In/Decode Compass ==
  note: Status Field can be one of the following:
      | L = low alarm
      | M= low warning
      | N = Normal
      | O = High Warning
      | P = High Alarm
      | C = Tuning analog circuit
  note: Compas NMEA- Raw data from the Compass
  Compass NMEA : Inport
  "ASCII Decode " : xpcseriallib/ASCII Decode   format=$PTNTHPR,%f,%c%f,%c%f,%c  nvars=7  vartypes={ }
  Bus Creator : BusCreator  Inputs=3
  Correct Heading Angle Magnetic to True North : Subsystem
  "FIFO ASCII read " : xpcseriallib/FIFO ASCII read   header={'$PTNTHPR'}  term=[13 10]  hold=Zero output if no new data  enable=off  maxsize=64  outputtype=8 bit uint null terminated  sampletime=-1
  Terminator{,1..3} (4 alike) : Terminator
  Compass data (3) : Outport
  wires:
  "FIFO ASCII read "/1 -> "ASCII Decode "/1
  Compass NMEA/1 -> "FIFO ASCII read "/1
  "ASCII Decode "/2 -> Terminator/1
  "ASCII Decode "/4 -> Terminator1/1
  "ASCII Decode "/6 -> Terminator2/1
  "ASCII Decode "/7 -> Terminator3/1
  Bus Creator/1 -> Compass data (3)/1  "Compass"
  "ASCII Decode "/3 -> Bus Creator/2  "Pitch"
  "ASCII Decode "/5 -> Bus Creator/3  "Roll"
  "ASCII Decode "/1 -> Correct Heading Angle Magnetic to True North/1(Heading Mag)  "Heading"
  Correct Heading Angle Magnetic to True North/1(Heading True) -> Bus Creator/1  "Heading"

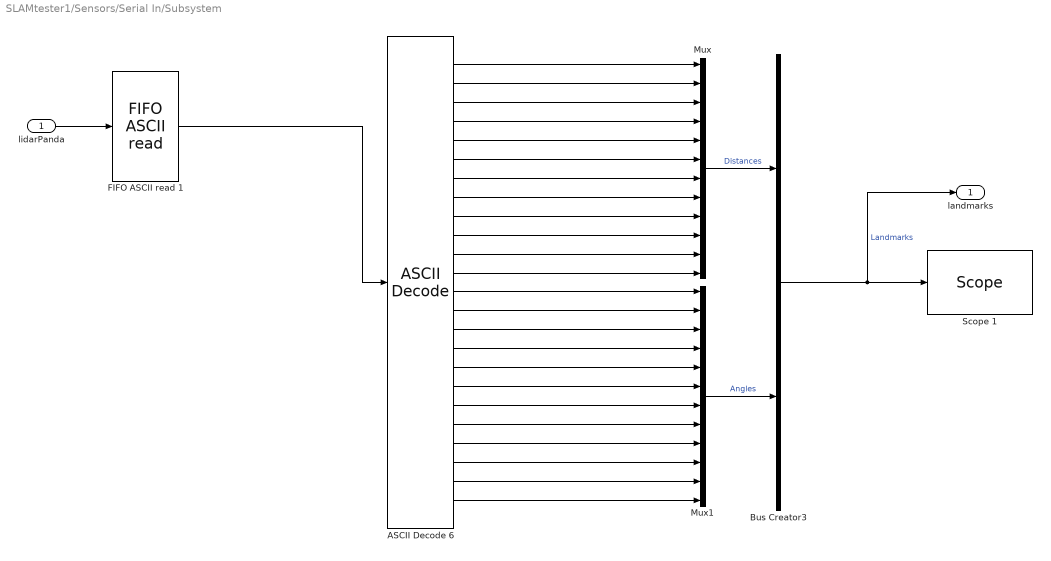
== system SLAMtester1/Sensors/Serial In/Subsystem ==
  lidarPanda : Inport
  ASCII Decode 6 : xpcseriallib/ASCII Decode   format=A:%f B:%f C:%f D:%f E:%f F:%f G:%f H:%f I:%f J:%f k:%f L:%f M:%d N:%d O:%d P:%d Q:%d R:%d S:%d T:%d U:%d V:%d W:%d X:%d  nvars=24  vartypes={}
  Bus Creator3 : BusCreator  Inputs=2
  FIFO ASCII read 1 : xpcseriallib/FIFO ASCII read   header={'A:'}  term=[13 10]  hold=Zero output if no new data  enable=off  maxsize=1024  outputtype=8 bit uint null terminated  sampletime=0.1
  Mux : Mux  Inputs=12
  Mux1 : Mux  Inputs=12
  Scope 1 : slrtlib/Displays and Logging/Scope   scopeno=2  scopetype=Host  autostart=on  viewmode=Graphical redraw  formatstr='%15.6f'  grid=on  ylimits=[0,0]  nosamples=24  noprepostsamples=0  interleave=1  triggermode=FreeRun  triggersignal=1  trigsignalfromport=off  triggerlevel=0.0  triggerslope=Either  triggerscope=1  triggersample=0  filename=data.dat  mode=Lazy  writesize=512  autorestart=off  dynamicfilemode=off  maxwritefilesize=512*1024^2
  landmarks : Outport
  wires:
  FIFO ASCII read 1/1 -> ASCII Decode 6/1
  Mux/1 -> Bus Creator3/1  "Distances"
  ASCII Decode 6/3 -> Mux/3
  ASCII Decode 6/4 -> Mux/4
  ASCII Decode 6/5 -> Mux/5
  ASCII Decode 6/9 -> Mux/9
  ASCII Decode 6/11 -> Mux/11
  ASCII Decode 6/8 -> Mux/8
  ASCII Decode 6/6 -> Mux/6
  ASCII Decode 6/10 -> Mux/10
  ASCII Decode 6/7 -> Mux/7
  ASCII Decode 6/12 -> Mux/12
  ASCII Decode 6/14 -> Mux1/2
  ASCII Decode 6/17 -> Mux1/5
  ASCII Decode 6/13 -> Mux1/1
  ASCII Decode 6/15 -> Mux1/3
  ASCII Decode 6/18 -> Mux1/6
  ASCII Decode 6/19 -> Mux1/7
  ASCII Decode 6/16 -> Mux1/4
  ASCII Decode 6/20 -> Mux1/8
  ASCII Decode 6/21 -> Mux1/9
  ASCII Decode 6/22 -> Mux1/10
  ASCII Decode 6/23 -> Mux1/11
  ASCII Decode 6/24 -> Mux1/12
  Mux1/1 -> Bus Creator3/2  "Angles"
  Bus Creator3/1 -> landmarks/1, Scope 1/1  "Landmarks"
  lidarPanda/1 -> FIFO ASCII read 1/1
  ASCII Decode 6/2 -> Mux/2
  ASCII Decode 6/1 -> Mux/1

== system SLAMtester1/Sinks/actuators/analog output ==
  Compass Heading : Inport
  Control Signals : Inport  Port=2
  Analog output : speedgoatlib_IO102/Analog output  id=1  channels=[1,2,3,4]  range=2  ts=0.1  pciSlot=-1
  Ground : Ground
  Subsystem : Subsystem
  wires:
  Subsystem/1(Propulsion) -> Analog output/1
  Subsystem/2(Steering) -> Analog output/2
  Control Signals/1 -> Subsystem/2(Control Signals)
  Compass Heading/1 -> Subsystem/1(Compass Heading)
  Ground/1 -> Analog output/4, Analog output/3

== system SLAMtester1/Sinks/actuators/digital output ==
  Digital Out : Inport
  Digital output : speedgoatlib_IO102/Digital output  id=1  channels=[1,2,3,4,5,6,7,8]  ts=0.1  pciSlot=-1
  Ground : Ground
  Terminator : Terminator
  wires:
  Digital Out/1 -> Terminator/1
  Ground/1 -> Digital output/1, Digital output/2, Digital output/3, Digital output/4, Digital output/5, Digital output/6, Digital output/7, Digital output/8

== system SLAMtester1/Sensors/Serial In/Decode Compass/Correct Heading Angle Magnetic to True North ==
  Heading Mag : Inport
  Magnetic to True North Conversion : MATLAB Function  TreatAsAtomicUnit=on
  Heading True : Outport
  wires:
  Magnetic to True North Conversion/1(HeadingT) -> Heading True/1  "Heading"
  Heading Mag/1 -> Magnetic to True North Conversion/1(HeadingM)

== system SLAMtester1/Sinks/actuators/analog output/Subsystem ==
  Compass Heading : Inport
  Control Signals : Inport  Port=2
  Bus Selector : BusSelector  OutputSignals=RPM,Desired Heading
  Heading Controller : Subsystem
  Propulsion Controller : Subsystem
  Propulsion : Outport
  Steering : Outport  Port=2
  wires:
  Control Signals/1 -> Bus Selector/1
  Bus Selector/1 -> Propulsion Controller/1(RPM)  "<RPM>"
  Propulsion Controller/1(Propulsion) -> Propulsion/1
  Bus Selector/2 -> Heading Controller/1(Heading Desired)  "<Desired Heading>"
  Compass Heading/1 -> Heading Controller/2(Compass Heading)
  Heading Controller/1(Steering) -> Steering/1

== system SLAMtester1/Sinks/actuators/analog output/Subsystem/Heading Controller ==
  Heading Desired : Inport
  Compass Heading : Inport  Port=2
  Gain : Gain  Gain=-0.05
  MATLAB Function : MATLAB Function  TreatAsAtomicUnit=on
  Saturation : Saturate  UpperLimit=5  LowerLimit=0
  Sum : Sum  Inputs=++|
  Voltage Nuetral : Constant  Value=2.5
  Steering : Outport
  wires:
  Compass Heading/1 -> MATLAB Function/2(CompassHeading)
  Heading Desired/1 -> MATLAB Function/1(HeadingDesired)
  MATLAB Function/1(steering) -> Gain/1
  Gain/1 -> Sum/2
  Voltage Nuetral/1 -> Sum/1
  Sum/1 -> Saturation/1
  Saturation/1 -> Steering/1

== system SLAMtester1/Sinks/actuators/analog output/Subsystem/Propulsion Controller ==
  RPM : Inport
  Saturation : Saturate  UpperLimit=5  LowerLimit=0
  Sum : Sum  Inputs=++|
  Voltage Neutral : Constant  Value=2.5
  Volts / RPM : Gain  Gain=2.5/6000
  Propulsion : Outport
  wires:
  RPM/1 -> Volts / RPM/1
  Volts / RPM/1 -> Sum/2
  Voltage Neutral/1 -> Sum/1
  Sum/1 -> Saturation/1
  Saturation/1 -> Propulsion/1

== matlab function SLAMtester1/Sinks/actuators/analog output/Subsystem/Heading Controller/MATLAB Function ==
  data: HeadingDesired input; steering output; CompassHeading input
function steering = CalcSteering(HeadingDesired, CompassHeading)

%Written by Anderson Lebbad on July 19, 2013
%Last Edited: Anderson Lebbad on August 14, 2013
%   Simplified using mod division

%Calculates the difference between the desired and current heading to be
%used for steering


%difference is calculated in the range of -180 to 180
steering = mod(HeadingDesired - CompassHeading, 360);
if steering > 180
    steering = steering - 360;
end

== matlab function SLAMtester1/Main FSM/landmarks_load ==
  data: roll output; dist input; ang input; imu input; gps input; motor input
function roll  = landmarks_load(dist,ang,imu,gps,motor)
%%[time, dtime, r_wheel desired speed, r_wheel measured speed, 
%l_wheel desired speed, l_wheel measured speed];

%% Init block run this block only once.

persistent timestep particles; 
timestep=2;
num_particles = 50;
% % The maximum distance from which our sensor can sense a landmark
max_read_distance = 5;
min_read_distance = 0.3;
min_read_angle = -22*pi/180; %radians- maximum read angle
max_read_angle = 22*pi/180;
% The initial starting position of the robot
avg_robot_position = [0;      % x %Use UTM coordinates from GPS 
                 0;     % y
                 0];  % rotation               
% The Gaussian variance of the movement commands
movement_variance = [.1;   % Left wheel
                     .1]; % Right_wheel
M = [movement_variance(1), 0.0;
     0.0, movement_variance(2)];
measurement_variance = [0.01;    % Distance
                        0.01];   % Angle
R = [measurement_variance(1), 0.0;
     0.0, measurement_variance(2)];
 default_importance=0.0000001; 
 pos_history = [];
 
%  if ~isempty(particles)
    % Create the particles and initialize them all to be in the same initial
    % position.
    %  field1='w';            value1=1.0/num_particles;
    %  field2='position';       value2=avg_robot_position;
    %  field3='num_landmarks';       value3=0;
    %  field4='lm_weight';       value4=1.0/num_particles;
    %  part = struct(field1,value1,field2,value2,field3,value3,field4,value4);
    %  particles=repmat(part,50);
    particles=repmat(struct('w',1.0/num_particles,'position',avg_robot_position,'num_landmarks',zeros(1,300),'lm_weight',repmat(1.0/num_particles,2,15),'landmarks',repmat(struct('pos',zeros(1,2),'E',zeros(6,6),'counter',0,'size_E',zeros(1,2)),1,15)),1,50);
    avg_robot_position = average_pos(particles,num_particles);
%  end
 
 
 

%% Load data
landmark1 = [dist(1),ang(1)];
landmark2 = [dist(2),ang(2)];
landmark3 = [dist(3),ang(3)];
landmark4 = [dist(4),ang(4)];
landmark5 = [dist(5),ang(5)];
landmark6 = [dist(6),ang(6)];
landmark7 = [dist(7),ang(7)];
landmark8 = [dist(8),ang(8)];
landmark9 = [dist(9),ang(9)];
landmark10 = [dist(10),ang(10)];
landmark11 = [dist(11),ang(11)];
landmark12 = [dist(12),ang(12)];

roll=imu(1);
pitch=imu(2);
yaw=imu(3);

dt=0;
r_wheel_des= 0;
r_wheel_mes= 0;
l_wheel_des= 0;
l_wheel_mes= 0;


  %% Move the actual particles
  % Needs replaced for new model.
  
  
  for pIdx = 1:num_particles
      
      %particles(pIdx).position = MoveMrT(particles(pIdx).position, [data(timestep,3) data(timestep,5)],movement_variance,data(timestep,2));
      %newpos = MoveMrT(pos, movement, variance,dt
    l_wheel_des    = normrnd(l_wheel_des, movement_variance(1));
    r_wheel_des = normrnd(r_wheel_des, movement_variance(2));
    wheel_radius = 0.04445; %m 
    wheel_base = 0.3175; %m
  
  %wheel velocities
    vel_right = r_wheel_des*wheel_radius;
    vel_left = l_wheel_des*wheel_radius;
  
    v_robot = (vel_right+vel_left)/2; %forward velocity of robot m/s
    omega_robot = (vel_left-vel_right)/wheel_base; %angular velocity of robot
  
    x_dot = sin(particles(pIdx).position(3))*v_robot;
    y_dot = cos(particles(pIdx).position(3))*v_robot;
    
    particles(pIdx).position(1) = particles(pIdx).position(1)+x_dot*dt;
    particles(pIdx).position(2) =  particles(pIdx).position(2)+y_dot*dt;
    particles(pIdx).position(3) = particles(pIdx).position(3)+omega_robot*dt;
      
  end
  
  
  z_real=[0;0];
  %%
  % Try to take a reading from each landmark
  doResample = false;
% The input got from landmarks
  collected_data=[-0.119955307371067,2.31463298709723,0.270433587697713,2.06920493403612,0.270712733973202,2.06936515522061,-0.119955307371067,2.31463298709723,0.270433587697713,2.06920493403612,0.270712733973202,2.06936515522061];
  [,cols,]=find(collected_data ~= 0);
  if (isempty(cols)==0)% if the cols is not empty
      doResample=true; %if there is new measurement, then resample particles
  end
  

  if (doResample==true)
      [r,c]=size(cols);
      shiva=1;
      for lIdx = 1:2:c %amount of visible landmarks
        real_landmark = [collected_data(1,lIdx),collected_data(1,lIdx+1)];
        % Take a real (noisy) measurement from the robot to the landmark
%         [z_real(:,lIdx), G(:,:,lIdx)] = getRealMeasurement(avg_robot_position, real_landmark, [0 0]);
%         function [z, H] = getRealMeasurement(pos, landmark_pos, observation_variance)
        
        landmark_angle=real_landmark(1);
        landmark_distance=real_landmark(2);

        % Compute the Jacobian of this measurement function
        q = landmark_distance^2.0;
    
        H = [-(real_landmark(1) - avg_robot_position(1))/sqrt(q), -(real_landmark(2) - avg_robot_position(2))/sqrt(q);
        (real_landmark(2) - avg_robot_position(2))/q,       -(real_landmark(1) - avg_robot_position(1))/q];


        z_real = [landmark_distance; landmark_angle];
%         read_distance(shiva) = landmark_distance;
%         read_angle(shiva)    = landmark_angle;
      end
      
      
      
      %% Actual for each particle calculation.
      
      
      for pIdx = 1:num_particles               
%           
% %           particles(pIdx).lm_weight=[];
% %           clear z_p H Q
          for j=1:particles(pIdx).num_landmarks(timestep-1)
%                 
% %               [z_p(:,j), H(:,:,j)] = getMeasurement(particles(pIdx).position, particles(pIdx).landmarks(j).pos, [0 0]);
% %               function [z, H] = getMeasurement(pos, landmark_pos, observation_variance)
                observation_variance=[0 0];
                vector_to_landmark = [particles(pIdx).landmarks(j).pos(1) - particles(pIdx).position(1); particles(pIdx).landmarks(j).pos(2) - particles(pIdx).position(2)];
                landmark_distance = norm(vector_to_landmark);
                %   landmark_distance = landmark_distance + normrnd(0, observation_variance(1)*.25);
                landmark_distance = landmark_distance;

                 % Compute the angle from the given pos to the landmark
                landmark_angle = atan2(vector_to_landmark(1), vector_to_landmark(2))-particles(pIdx).position(3);
                %   landmark_angle = landmark_angle + normrnd(0, observation_variance(2)*.25);
                landmark_angle = landmark_angle;

                  % Compute the Jacobian of this measurement function
                q = landmark_distance^2.0;
                %   H = [-(landmark_pos(1) - pos(1))/sqrt(q), -(landmark_pos(2) - pos(2))/sqrt(q), 0.0;
                %         (landmark_pos(2) - pos(2))/q,       -(landmark_pos(1) - pos(1))/q,      -1.0;
                %         0.0,                                0.0,                               1.0];

                H = [-(particles(pIdx).landmarks(j).pos(1) - particles(pIdx).position(1))/landmark_distance, -(particles(pIdx).landmarks(j).pos(2) - particles(pIdx).position(2))/landmark_distance;
                        (particles(pIdx).landmarks(j).pos(2) - particles(pIdx).position(2))/q,       -(particles(pIdx).landmarks(j).pos(1) - particles(pIdx).position(1))/q];
 
                z_p = [landmark_distance; 
                    landmark_angle];
% 
              for measured_lm=1:size(z_real,2) 
                residual = z_real(:,measured_lm) - z_p(:,j);
                Q=zeros(size(R));
                E=zeros(particles(pIdx).landmarks(j).size_E);
                E=particles(pIdx).landmarks(j).E(1:particles(pIdx).landmarks(j).size_E(1,1),1:particles(pIdx).landmarks(j).size_E(1,2));
%                 E=particles(pIdx).landmarks(j).E()

                Q(:,:,j) = H(:,:,j)' * E * H(:,:,j) + R;             
                particles(pIdx).lm_weight(measured_lm,j) = particles(pIdx).w * norm(2*pi*Q(:,:,j)).^(-1/2)*exp(-1/2*(residual)'*inv(Q(:,:,j))*(residual));
              end
          end
          
                    %probably going to delete this hold on for now
          %           particles(pIdx).lm_weight(particles(pIdx).num_landmarks(timestep-1)+1) = 0.09; %importance factor, new feature
          particles(pIdx).num_landmarks(timestep)=particles(pIdx).num_landmarks(timestep-1);
          %           clear c_hat
          
          cost_table=zeros(size(z_real,2),particles(pIdx).num_landmarks(timestep-1));
          cost_table(1:size(z_real,2),1:particles(pIdx).num_landmarks(timestep-1))=particles(pIdx).lm_weight(1:particles(pIdx).num_landmarks(timestep-1));
% need to work on this          cost_table(1:size(z_real,2),particles(pIdx).num_landmarks(timestep-1)+1:particles(pIdx).num_landmarks(timestep-1)+size(z_real,2))=default_importance*eye(size(z_real,2));
          if(isempty(max(max(cost_table)))) particles(pIdx).w=0;
%           else particles(pIdx).w=max(max(cost_table));
          end
          [~, idx_hold]=max(cost_table,[],1); %this is the max correseponding for each measurement
          for i=1:size(cost_table,2)
             idx_zero=setdiff([1:size(cost_table,1)],idx_hold(i));
             cost_table(idx_zero,i)=0;
          end

          
          
          
          
          
          
          
          
      end % End of pIdx = 1:num_particles
      
      
      
      
      
      
      
      
      
      
      
      
      
      
      
      
      
      
      
      
      
      
      
      
      
%% the end for the condition to make sure if there is no measurements to not alculate things.      
  end
  
  
  
  
  
  
  
  
  
  
  
  
  
  
        
     




y= r_wheel_des;


end


function avg_robot_position = average_pos(particles,num_particles)
 xsiva=0;
 ysiva=0;
 rotsiva=0;
 
 for siva=1:num_particles
     xsiva=xsiva+particles(siva).position(1);
     ysiva=ysiva+particles(siva).position(2);
     rotsiva=rotsiva+particles(siva).position(3);
 end

avg_robot_position = [xsiva/num_particles; ysiva/num_particles; rotsiva/num_particles];

end

== matlab function SLAMtester1/Sensors/Serial In/Decode Compass/Correct Heading Angle Magnetic to True North/Magnetic to True North Conversion ==
  data: HeadingM input; HeadingT output
function HeadingT = fcn(HeadingM)
% This block supports the Embedded MATLAB subset.
% See the help menu for details. 

HeadingT=HeadingM+180-12.3; %180 was added since compass was rotated when
                            %it was relocated.

if HeadingT>360
    HeadingT=HeadingT-360;
elseif HeadingT<0;
    HeadingT=HeadingT+360;
end

== matlab function SLAMtester1/Parameters/GPS Points/GPS Selector ==
  data: course input; ssGate output; rtnIn input; ssGateA input; colorA input; obstNavStartA input; obstNavEndA input; acouLocA input; dockA input; ssGateB input; colorB input; obstNavStartB input; obstNavEndB input; acouLocB input; dockB input; ssGateT input; colorT input; obstNavStartT input; obstNavEndT input; acouLocT input; dockT input; color output; obstNavStart output; obstNavEnd output; acouLoc output; dock output; rtnOut output
function [ssGate,color,obstNavStart,obstNavEnd,acouLoc,dock,rtnOut] = ...
    GPSselector(course,rtnIn,...
    ssGateA,colorA,obstNavStartA,obstNavEndA,acouLocA,dockA,...
    ssGateB,colorB,obstNavStartB,obstNavEndB,acouLocB,dockB,...
    ssGateT,colorT,obstNavStartT,obstNavEndT,acouLocT,dockT)

%Written by: Anderson Lebbad on July 18, 2013
%Last Edited: Edward Zhu on June
%   Data type mismatch addressed
%   Character conversion redundant

%Selects GPS Points to use based on input Course

%Check value of CourseStr and pass inputs accordingly

switch course
    case uint8('A')
        ssGate = ssGateA;
        color = colorA;
        obstNavStart = obstNavStartA;
        obstNavEnd = obstNavEndA;
        acouLoc = acouLocA;
        dock = dockA;
        rtnOut = rtnIn;
        
    case uint8('B')
        ssGate = ssGateB;
        color = colorB;
        obstNavStart = obstNavStartB;
        obstNavEnd = obstNavEndB;
        acouLoc = acouLocB;
        dock = dockB;
        rtnOut = rtnIn;
        
    otherwise
        ssGate = ssGateT;
        color = colorT;
        obstNavStart = obstNavStartT;
        obstNavEnd = obstNavEndT;
        acouLoc = acouLocT;
        dock = dockT;
        rtnOut = rtnIn;
end

== matlab function SLAMtester1/Parameters/Task Selector/Message Composer ==
  data: taskStrInit input; taskStrAdj output
function taskStrAdj = composeMessage(taskStrInit)
%Written by Anderson Lebbad on August 9, 2013
%Last Edited: Edward Zhu on June 2, 2014

%This function adjusts the length of a vector to a set value by filling
%the remaining space with 0's. This is necessary for data store objects
%that have a fixed size for the memory allocation, but a variable length
%input.

%Length of message packet
strLength = 8;

%Size of text in message
taskStrLength = size(taskStrInit,1);

%Pad end of text with zeros
taskStrAdj = [taskStrInit' zeros(1,strLength-taskStrLength)];

== matlab function SLAMtester1/Parameters/Task Selector/Message Composer1 ==
  data: taskStrInit input; taskStrAdj output
function taskStrAdj = composeMessage(taskStrInit)
%Written by Anderson Lebbad on August 9, 2013
%Last Edited: Edward Zhu on June 2, 2014

%This function adjusts the length of a vector to a set value by filling
%the remaining space with 0's. This is necessary for data store objects
%that have a fixed size for the memory allocation, but a variable length
%input.

%Length of message packet
strLength = 8;

%Size of text in message
taskStrLength = size(taskStrInit,1);

%Pad end of text with zeros
taskStrAdj = [taskStrInit' zeros(1,strLength-taskStrLength)];
